simulink model "AC_motor_4"  (R2024b)
settings: Solver=FixedStepAuto  StartTime=0.0  StopTime=Tsimulation  FixedStep=Ts  RelTol=1e-3  EnableMultiTasking=on
values from neighbouring files (symbols this model uses):
  fb = 50    [AIR_Generation.m]    (also in Find_Best_Noizz.m; input_AIR80B4_3_broken_rods.m)
  J = 0.0226    [AIR_Generation.m]    (also in Find_Best_Noizz.m; input_AIR80B4_3_broken_rods.m)
  Lm = Ls - Lls    [Calculate_Basic.m]    (also in Find_Best_Noizz.m = 0.401; input_AIR80B4_3_broken_rods.m = 0.401)
  Lr = Ls    [Calculate_Basic.m]    (also in Find_Best_Noizz.m = 0.414; Run_Short_Circuit_Simulation.m = Lr*((nturns_phase-fscnturns)/nturns_phase)^2; input_AIR80B4_3_broken_rods.m = Lr*((nturns_phase-fscnturns)/nturns_phase)^2)
  Ls = 1 / 2 / pi / fb * Vph / In / (sqrt(1 - cosfi ^ 2) - cosfi * Sn / Sk)    [Calculate_Basic.m]    (also in Find_Best_Noizz.m = 0.414; Run_Short_Circuit_Simulation.m = Ls*((nturns_phase-fscnturns)/nturns_phase)^2; input_AIR80B4_3_broken_rods.m = Ls*((nturns_phase-fscnturns)/nturns_phase)^2)
  P = data{i, 2} / 2    [AIR_Generation.m]    (also in Find_Best_Noizz.m = 2; input_AIR80B4_3_broken_rods.m = 2)
  Rr = 1 / 3 * (Power + dPm) / Ikn ^ 2 / In ^2 / (1 - Sn)    [Calculate_Basic.m]    (also in Find_Best_Noizz.m = 1.274; Run_Short_Circuit_Simulation.m = Rr*((nturns_phase-fscnturns)/nturns_phase)^2; input_AIR80B4_3_broken_rods.m = Rr*((nturns_phase-fscnturns)/nturns_phase)^2)
  Rs = 1.5 * Vph ^ 2 * (1 - Sn) / C1 / (1 + C1 / Sk) / mk / (Power + dPm)    [Calculate_Basic.m]    (also in Find_Best_Noizz.m = 3.523; Run_Short_Circuit_Simulation.m = Rs*((nturns_phase-fscnturns)/nturns_phase); input_AIR80B4_3_broken_rods.m = Rs*((nturns_phase-fscnturns)/nturns_phase))
  Ts = 2e-5    (= 2e-05)    [AIR_Generation.m]    (also in Find_Best_Noizz.m; input_AIR80B4_3_broken_rods.m)
  Tswrite = 0.24e-3    (= 0.00024)    [AIR_Generation.m]    (also in Find_Best_Noizz.m; input_AIR80B4_3_broken_rods.m)
  Vph = Un / sqrt(3)    [AIR_Generation.m]    (also in Find_Best_Noizz.m = 380/sqrt(3); input_AIR80B4_3_broken_rods.m = 380/sqrt(3))
libraries: simulink x6
settings Model: Creator=srikanth  LastModifiedBy=rusla
settings SolverCC: AlgebraicLoopSolver=TrustRegion
settings DataIOCC: SignalLoggingSaveFormat=ModelDataLogs
settings OptimizationCC: ExpressionDepthLimit=2147483647  LifeSpan=inf  SimCompilerOptimization=on
settings DebuggingCC: UnderspecifiedInitializationDetection=Classic  MergeDetectMultiDrivingBlocksExec=none  FcnCallInpInsideContextMsg=warning  UnconnectedInputMsg=warning  UnconnectedOutputMsg=warning  UnconnectedLineMsg=warning  StateNameClashWarn=warning  SFUnexpectedBacktrackingDiag=warning  SFNoUnconditionalDefaultTransitionDiag=warning  SFExecutionAtInitializationDiag=none  ArithmeticOperatorsInVariantConditions=warning
settings HardwareCC: ProdBitPerPointer=32  ProdBitPerSizeT=32  ProdBitPerPtrDiffT=32  ProdLargestAtomicFloat=None  ProdIntDivRoundTo=Undefined  ProdEndianess=Unspecified  ProdWordSize=32  ProdHWDeviceType=32-bit Generic
settings ModelReferenceCC: PropagateSignalLabelsOutOfModel=off
settings SFSimCC: SimUseLocalCustomCode=off  CustomCodeUndefinedFunction=UseInterfaceOnly
settings RTWCC: RTWUseLocalCustomCode=off  GPUComputeCapability=3.5
settings CodeAppCC: StateflowObjectComments=on
settings GRTTargetCC: TargetLangStandard=C89/C90 (ANSI)  CombineOutputUpdateFcns=off  GRTInterface=on
settings ConfigComp: CovMetricSettings=dw  CovSaveCumulativeToWorkspaceVar=on  CovSaveSingleToWorkspaceVar=on  CovExternalEMLEnable=off

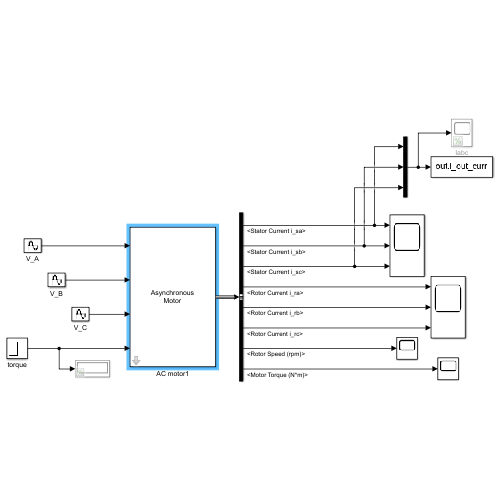
[thumbnail: Simulink's stored preview of the top-level diagram]
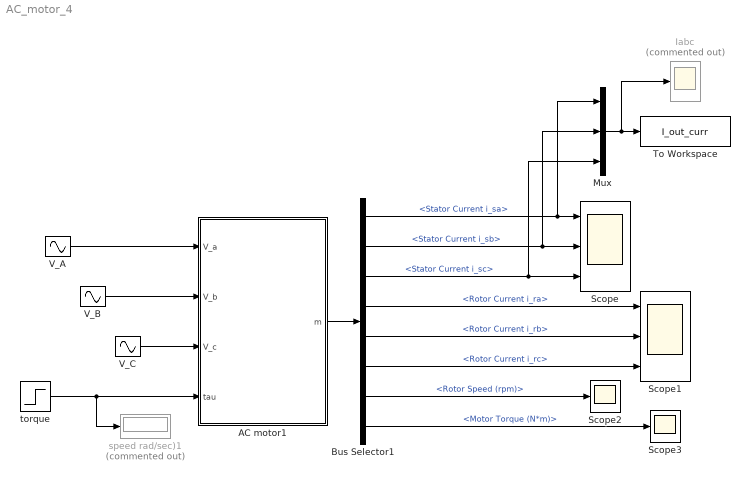
== system AC_motor_4 ==
  AC motor1 : Subsystem  mask{Rs=Rs, Ls=Ls, Rr=Rr, Lr=Lr, Lm=Lm, J=J, P=P*2}
      mask prompts: Rs "Stator Resistance  Rs [Ohm] :"; Ls "Stator Inductance Ls [H] :"; Rr "Rotor Resistance Rr [Ohm] :"; Lr "Rotor Inductance Lr [H] :"; Lm "Mutual Inductance Lm [H] :"; J "Rotor Inertia J [Kg/m^2] :"; P "Number of Poles p :"
      mask Display: fprintf('Asynchronous\nMotor')
  Bus Selector1 : BusSelector  OutputSignals=Stator.Stator Current i_sa,Stator.Stator Current i_sb,Stator.Stator Current i_sc,Rotor.Rotor Current i_ra,Rotor.Rotor Current i_rb,Rotor.Rotor Current i_rc,Mechanical.Rotor Speed (rpm),Mechanical.Motor Torque (N*m)
  Iabc : Scope  Commented=on
  Mux : Mux  Inputs=3
  Scope : Scope  NumInputPorts=3
  Scope1 : Scope  NumInputPorts=3
  Scope2 : Scope
  Scope3 : Scope
  To Workspace : ToWorkspace  VariableName=I_out_curr  SaveFormat=Structure With Time  SampleTime=Tswrite
  V_A : Sin  Amplitude=Vph  Frequency=2*pi*fb  SampleTime=Ts
  V_B : Sin  Amplitude=Vph  Frequency=2*pi*fb  Phase=-2*pi/3  SampleTime=Ts
  V_C : Sin  Amplitude=Vph  Frequency=2*pi*fb  Phase=2*pi/3  SampleTime=Ts
  speed rad/sec)1 : Display  Commented=on
  torque : Step  Time=2  After=2.3  SampleTime=0
  wires:
  torque/1 -> AC motor1/4(tau), speed rad/sec)1/1
  V_A/1 -> AC motor1/1(V_a)
  V_B/1 -> AC motor1/2(V_b)
  V_C/1 -> AC motor1/3(V_c)
  Bus Selector1/2 -> Mux/2, Scope/2  "<Stator Current i_sb>"
  Bus Selector1/3 -> Mux/3, Scope/3  "<Stator Current i_sc>"
  Bus Selector1/5 -> Scope1/2  "<Rotor Current i_rb>"
  Bus Selector1/8 -> Scope3/1  "<Motor Torque (N*m)>"
  Bus Selector1/4 -> Scope1/1  "<Rotor Current i_ra>"
  Bus Selector1/7 -> Scope2/1  "<Rotor Speed (rpm)>"
  Bus Selector1/6 -> Scope1/3  "<Rotor Current i_rc>"
  Bus Selector1/1 -> Mux/1, Scope/1  "<Stator Current i_sa>"
  Mux/1 -> Iabc/1, To Workspace/1
  AC motor1/1(m) -> Bus Selector1/1

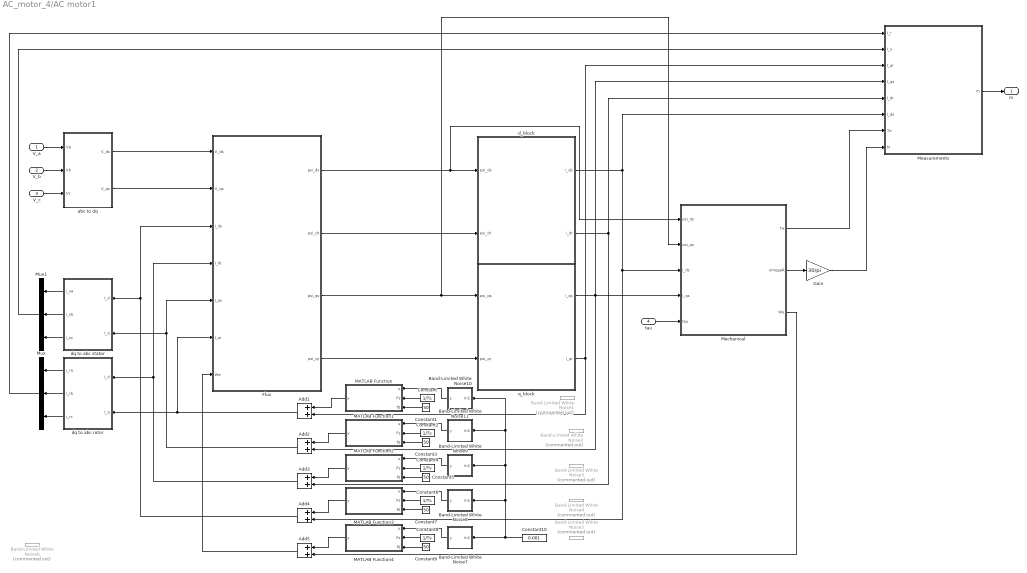
== system AC_motor_4/AC motor1 ==
  V_a : Inport
  V_b : Inport  Port=2
  V_c : Inport  Port=3
  tau : Inport  Port=4
  Add{1..5} (5 alike) : Sum
  Band-Limited White Noise1 : simulink/Sources/Band-Limited White Noise  Commented=on  Cov=[0.00001]  Ts=Ts  seed=[426526]
  Band-Limited White Noise10 : Subsystem  mask{Ts=Ts, seed=[426526]}
      mask prompts: Ts "Sample time:"
  Band-Limited White Noise11 : Subsystem  mask{Ts=Ts, seed=[921372]}
      mask prompts: Ts "Sample time:"
  Band-Limited White Noise2 : simulink/Sources/Band-Limited White Noise  Commented=on  Cov=[0.00001]  Ts=Ts  seed=[921372]
  Band-Limited White Noise3 : simulink/Sources/Band-Limited White Noise  Commented=on  Cov=[0.00001]  Ts=Ts  seed=[152264]
  Band-Limited White Noise4 : simulink/Sources/Band-Limited White Noise  Commented=on  Cov=[0.00001]  Ts=Ts  seed=[675373]
  Band-Limited White Noise5 : simulink/Sources/Band-Limited White Noise  Commented=on  Cov=[0.00001]  Ts=Ts  seed=[285858]
  Band-Limited White Noise6 : simulink/Sources/Band-Limited White Noise  Commented=on  Cov=[0.00001]  Ts=Ts  seed=[285858]
  Band-Limited White Noise7 : Subsystem  mask{Ts=Ts, seed=[285858]}
      mask prompts: Ts "Sample time:"
  Band-Limited White Noise8 : Subsystem  mask{Ts=Ts, seed=[675373]}
      mask prompts: Ts "Sample time:"
  Band-Limited White Noise9 : Subsystem  mask{Ts=Ts, seed=[152264]}
      mask prompts: Ts "Sample time:"
  Constant{,2,4,6,8} (5 alike) : Constant  Value=1/Ts
  Constant{1,3,5,7,9} (5 alike) : Constant  Value=50
  Constant10 : Constant  Value=0.001
  Flux : Subsystem
  Gain : Gain  Gain=30/pi
  MATLAB Function : MATLAB Function  TreatAsAtomicUnit=on
  MATLAB Function1 : MATLAB Function  TreatAsAtomicUnit=on
  MATLAB Function2 : MATLAB Function  TreatAsAtomicUnit=on
  MATLAB Function3 : MATLAB Function  TreatAsAtomicUnit=on
  MATLAB Function4 : MATLAB Function  TreatAsAtomicUnit=on
  Measurements : Subsystem
  Mechanical : Subsystem
  Mux : Mux  Inputs=3
  Mux1 : Mux  Inputs=3
  abc to dq : Subsystem
  d_block : Subsystem
  dq to abc rotor : Subsystem
  dq to abc stator : Subsystem
  q_block : Subsystem
  m : Outport
  wires:
  V_c/1 -> abc to dq/3(Vc)
  V_b/1 -> abc to dq/2(Vb)
  V_a/1 -> abc to dq/1(Va)
  abc to dq/1(V_ds) -> Flux/1(V_ds)
  abc to dq/2(V_qs) -> Flux/2(V_qs)
  dq to abc rotor/3(i_rc) -> Mux/3
  dq to abc rotor/1(i_ra) -> Mux/1
  dq to abc rotor/2(i_rb) -> Mux/2
  dq to abc stator/1(i_sa) -> Mux1/1
  dq to abc stator/2(i_sb) -> Mux1/2
  dq to abc stator/3(i_sc) -> Mux1/3
  Flux/3(psi_qs) -> q_block/1(psi_qs), Mechanical/2(psi_qs)
  Flux/4(psi_qr) -> q_block/2(psi_qr)
  Flux/2(psi_dr) -> d_block/2(psi_dr)
  Flux/1(psi_ds) -> d_block/1(psi_ds), Mechanical/1(psi_ds)
  tau/1 -> Mechanical/5(tau)
  q_block/1(i_qs) -> Add2/2, Measurements/4(I_qs), Mechanical/4(i_qs)
  d_block/1(i_ds) -> Add4/2, Mechanical/3(i_ds), Measurements/6(I_ds)
  Mechanical/3(We) -> Add5/2
  Mechanical/2(omegaR) -> Gain/1
  d_block/2(i_dr) -> Add3/2, Measurements/5(I_dr)
  q_block/2(i_qr) -> Add1/2, Measurements/3(I_qr)
  Measurements/1(m) -> m/1
  Gain/1 -> Measurements/8(N)
  Mechanical/1(Te) -> Measurements/7(Te)
  Mux1/1 -> Measurements/2(I_s)
  Mux/1 -> Measurements/1(I_r)
  Band-Limited White Noise10/1(y) -> MATLAB Function/1(u)
  Add1/1 -> Flux/6(I_qr), dq to abc rotor/2(I_q)
  Add2/1 -> Flux/5(I_qs), dq to abc stator/2(I_q)
  Add3/1 -> Flux/4(I_dr), dq to abc rotor/1(I_d)
  Add4/1 -> Flux/3(I_ds), dq to abc stator/1(I_d)
  Add5/1 -> Flux/7(We)
  Band-Limited White Noise11/1(y) -> MATLAB Function1/1(u)
  Band-Limited White Noise9/1(y) -> MATLAB Function2/1(u)
  Band-Limited White Noise8/1(y) -> MATLAB Function3/1(u)
  Band-Limited White Noise7/1(y) -> MATLAB Function4/1(u)
  MATLAB Function/1(y) -> Add1/1
  Constant/1 -> MATLAB Function/2(Fs)
  Constant1/1 -> MATLAB Function/3(f0)
  Constant3/1 -> MATLAB Function1/3(f0)
  Constant2/1 -> MATLAB Function1/2(Fs)
  MATLAB Function1/1(y) -> Add2/1
  Constant4/1 -> MATLAB Function2/2(Fs)
  Constant5/1 -> MATLAB Function2/3(f0)
  MATLAB Function2/1(y) -> Add3/1
  Constant7/1 -> MATLAB Function3/3(f0)
  Constant6/1 -> MATLAB Function3/2(Fs)
  MATLAB Function3/1(y) -> Add4/1
  Constant8/1 -> MATLAB Function4/2(Fs)
  Constant9/1 -> MATLAB Function4/3(f0)
  MATLAB Function4/1(y) -> Add5/1
  Constant10/1 -> Band-Limited White Noise10/1(In1), Band-Limited White Noise11/1(In1), Band-Limited White Noise9/1(In1), Band-Limited White Noise8/1(In1), Band-Limited White Noise7/1(In1)

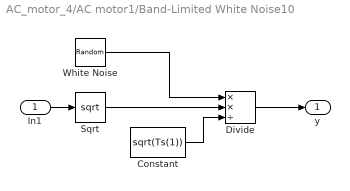
== system AC_motor_4/AC motor1/Band-Limited White Noise10 ==
  In1 : Inport
  Constant : Constant  Value=sqrt(Ts(1))
  Divide : Product  Inputs=**/
  Sqrt : Sqrt
  White Noise : RandomNumber  DisableCoverage=on  Seed=seed  SampleTime=Ts
  y : Outport
  wires:
  Sqrt/1 -> Divide/2
  In1/1 -> Sqrt/1
  Constant/1 -> Divide/3
  White Noise/1 -> Divide/1
  Divide/1 -> y/1

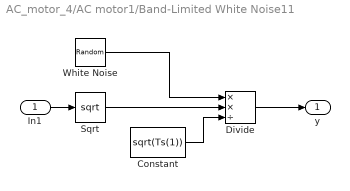
== system AC_motor_4/AC motor1/Band-Limited White Noise11 ==
  In1 : Inport
  Constant : Constant  Value=sqrt(Ts(1))
  Divide : Product  Inputs=**/
  Sqrt : Sqrt
  White Noise : RandomNumber  DisableCoverage=on  Seed=seed  SampleTime=Ts
  y : Outport
  wires:
  Divide/1 -> y/1
  White Noise/1 -> Divide/1
  Constant/1 -> Divide/3
  In1/1 -> Sqrt/1
  Sqrt/1 -> Divide/2

== system AC_motor_4/AC motor1/Band-Limited White Noise7 ==
  In1 : Inport
  Constant : Constant  Value=sqrt(Ts(1))
  Divide : Product  Inputs=**/
  Sqrt : Sqrt
  White Noise : RandomNumber  DisableCoverage=on  Seed=seed  SampleTime=Ts
  y : Outport
  wires:
  Divide/1 -> y/1
  White Noise/1 -> Divide/1
  Constant/1 -> Divide/3
  In1/1 -> Sqrt/1
  Sqrt/1 -> Divide/2

== system AC_motor_4/AC motor1/Band-Limited White Noise8 ==
  In1 : Inport
  Constant : Constant  Value=sqrt(Ts(1))
  Divide : Product  Inputs=**/
  Sqrt : Sqrt
  White Noise : RandomNumber  DisableCoverage=on  Seed=seed  SampleTime=Ts
  y : Outport
  wires:
  Sqrt/1 -> Divide/2
  In1/1 -> Sqrt/1
  Constant/1 -> Divide/3
  White Noise/1 -> Divide/1
  Divide/1 -> y/1

== system AC_motor_4/AC motor1/Band-Limited White Noise9 ==
  In1 : Inport
  Constant : Constant  Value=sqrt(Ts(1))
  Divide : Product  Inputs=**/
  Sqrt : Sqrt
  White Noise : RandomNumber  DisableCoverage=on  Seed=seed  SampleTime=Ts
  y : Outport
  wires:
  Divide/1 -> y/1
  White Noise/1 -> Divide/1
  Constant/1 -> Divide/3
  In1/1 -> Sqrt/1
  Sqrt/1 -> Divide/2

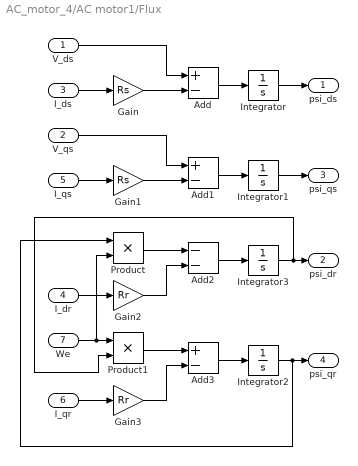
== system AC_motor_4/AC motor1/Flux ==
  V_ds : Inport
  V_qs : Inport  Port=2
  I_ds : Inport  Port=3
  I_dr : Inport  Port=4
  I_qs : Inport  Port=5
  I_qr : Inport  Port=6
  We : Inport  Port=7
  Add : Sum  Inputs=+-
  Add1 : Sum  Inputs=+-
  Add2 : Sum  Inputs=--
  Add3 : Sum  Inputs=+-
  Gain : Gain  Gain=Rs
  Gain1 : Gain  Gain=Rs
  Gain2 : Gain  Gain=Rr
  Gain3 : Gain  Gain=Rr
  Integrator{,1..3} (4 alike) : Integrator
  Product : Product
  Product1 : Product
  psi_ds : Outport
  psi_dr : Outport  Port=2
  psi_qs : Outport  Port=3
  psi_qr : Outport  Port=4
  wires:
  I_ds/1 -> Gain/1
  Gain/1 -> Add/2
  V_ds/1 -> Add/1
  Add/1 -> Integrator/1
  Integrator/1 -> psi_ds/1
  V_qs/1 -> Add1/1
  Gain1/1 -> Add1/2
  I_qs/1 -> Gain1/1
  Add1/1 -> Integrator1/1
  Integrator1/1 -> psi_qs/1
  Integrator2/1 -> Product/1, psi_qr/1
  Integrator3/1 -> Product1/2, psi_dr/1
  Add2/1 -> Integrator3/1
  Product/1 -> Add2/1
  I_dr/1 -> Gain2/1
  I_qr/1 -> Gain3/1
  Gain2/1 -> Add2/2
  We/1 -> Product/2, Product1/1
  Product1/1 -> Add3/1
  Gain3/1 -> Add3/2
  Add3/1 -> Integrator2/1

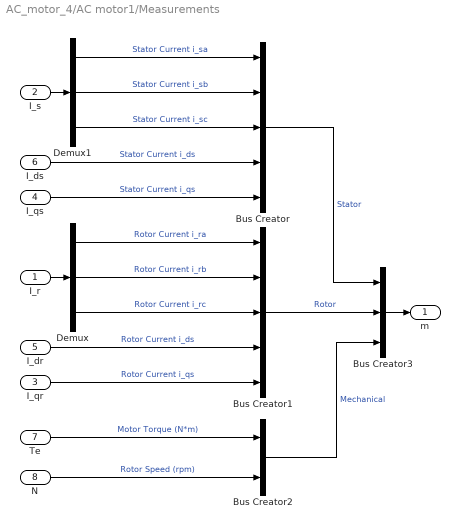
== system AC_motor_4/AC motor1/Measurements ==
  I_r : Inport
  I_s : Inport  Port=2
  I_qr : Inport  Port=3
  I_qs : Inport  Port=4
  I_dr : Inport  Port=5
  I_ds : Inport  Port=6
  Te : Inport  Port=7
  N : Inport  Port=8
  Bus Creator : BusCreator  Inputs=5
  Bus Creator1 : BusCreator  Inputs=5
  Bus Creator2 : BusCreator  Inputs=2
  Bus Creator3 : BusCreator  Inputs=3
  Demux : Demux  Outputs=3
  Demux1 : Demux  Outputs=3
  m : Outport
  wires:
  Bus Creator3/1 -> m/1
  Bus Creator/1 -> Bus Creator3/1  "Stator"
  Bus Creator1/1 -> Bus Creator3/2  "Rotor"
  Bus Creator2/1 -> Bus Creator3/3  "Mechanical"
  Te/1 -> Bus Creator2/1  "Motor Torque (N*m)"
  N/1 -> Bus Creator2/2  "Rotor Speed (rpm)"
  I_dr/1 -> Bus Creator1/4  "Rotor Current i_ds"
  I_qr/1 -> Bus Creator1/5  "Rotor Current i_qs"
  Demux/2 -> Bus Creator1/2  "Rotor Current i_rb"
  Demux/1 -> Bus Creator1/1  "Rotor Current i_ra"
  Demux/3 -> Bus Creator1/3  "Rotor Current i_rc"
  I_r/1 -> Demux/1
  Demux1/1 -> Bus Creator/1  "Stator Current i_sa"
  Demux1/2 -> Bus Creator/2  "Stator Current i_sb"
  Demux1/3 -> Bus Creator/3  "Stator Current i_sc"
  I_ds/1 -> Bus Creator/4  "Stator Current i_ds"
  I_qs/1 -> Bus Creator/5  "Stator Current i_qs"
  I_s/1 -> Demux1/1

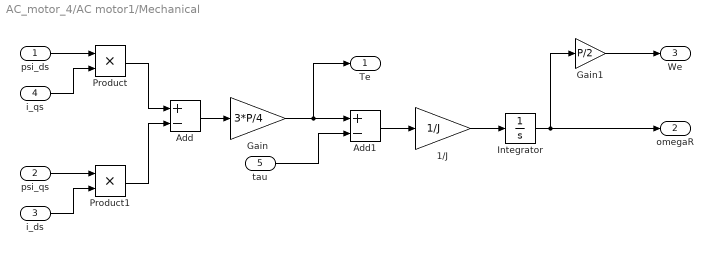
== system AC_motor_4/AC motor1/Mechanical ==
  psi_ds : Inport
  psi_qs : Inport  Port=2
  i_ds : Inport  Port=3
  i_qs : Inport  Port=4
  tau : Inport  Port=5
  1/J : Gain  Gain=1/J
  Add : Sum  Inputs=+-
  Add1 : Sum  Inputs=+-
  Gain : Gain  Gain=3*P/4
  Gain1 : Gain  Gain=P/2
  Integrator : Integrator
  Product : Product
  Product1 : Product
  Te : Outport
  omegaR : Outport  Port=2
  We : Outport  Port=3
  wires:
  psi_ds/1 -> Product/1
  i_qs/1 -> Product/2
  psi_qs/1 -> Product1/1
  i_ds/1 -> Product1/2
  Product/1 -> Add/1
  Product1/1 -> Add/2
  Add/1 -> Gain/1
  Gain/1 -> Add1/1, Te/1
  tau/1 -> Add1/2
  Add1/1 -> 1/J/1
  1/J/1 -> Integrator/1
  Gain1/1 -> We/1
  Integrator/1 -> Gain1/1, omegaR/1

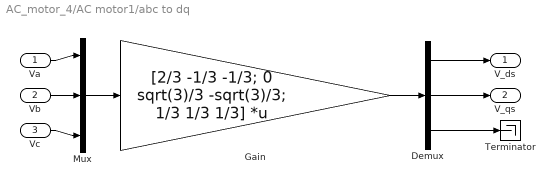
== system AC_motor_4/AC motor1/abc to dq ==
  Va : Inport
  Vb : Inport  Port=2
  Vc : Inport  Port=3
  Demux : Demux  Outputs=3
  Gain : Gain  Gain=[2/3 -1/3 -1/3; 0 sqrt(3)/3 -sqrt(3)/3; 1/3 1/3 1/3]  Multiplication=Matrix(K*u)
  Mux : Mux  Inputs=3
  Terminator : Terminator
  V_ds : Outport
  V_qs : Outport  Port=2
  wires:
  Va/1 -> Mux/1
  Vb/1 -> Mux/2
  Vc/1 -> Mux/3
  Mux/1 -> Gain/1
  Gain/1 -> Demux/1
  Demux/3 -> Terminator/1
  Demux/1 -> V_ds/1
  Demux/2 -> V_qs/1

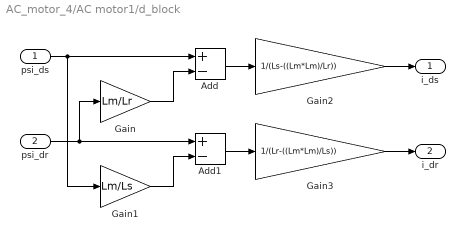
== system AC_motor_4/AC motor1/d_block ==
  psi_ds : Inport
  psi_dr : Inport  Port=2
  Add : Sum  Inputs=+-
  Add1 : Sum  Inputs=+-
  Gain : Gain  Gain=Lm/Lr
  Gain1 : Gain  Gain=Lm/Ls
  Gain2 : Gain  Gain=1/(Ls-((Lm*Lm)/Lr))
  Gain3 : Gain  Gain=1/(Lr-((Lm*Lm)/Ls))
  i_ds : Outport
  i_dr : Outport  Port=2
  wires:
  psi_ds/1 -> Add/1, Gain1/1
  Gain/1 -> Add/2
  Gain1/1 -> Add1/2
  psi_dr/1 -> Gain/1, Add1/1
  Gain2/1 -> i_ds/1
  Add/1 -> Gain2/1
  Add1/1 -> Gain3/1
  Gain3/1 -> i_dr/1

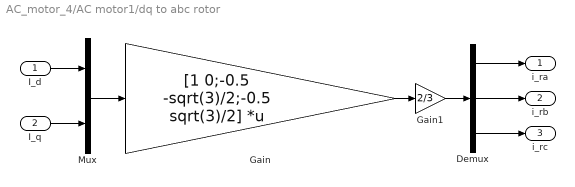
== system AC_motor_4/AC motor1/dq to abc rotor ==
  I_d : Inport
  I_q : Inport  Port=2
  Demux : Demux  Outputs=3
  Gain : Gain  Gain=[1 0;-0.5 -sqrt(3)/2;-0.5 sqrt(3)/2]  Multiplication=Matrix(K*u)
  Gain1 : Gain  Gain=2/3
  Mux : Mux  Inputs=2
  i_ra : Outport
  i_rb : Outport  Port=2
  i_rc : Outport  Port=3
  wires:
  Gain/1 -> Gain1/1
  Demux/1 -> i_ra/1
  I_q/1 -> Mux/2
  Demux/2 -> i_rb/1
  Mux/1 -> Gain/1
  I_d/1 -> Mux/1
  Gain1/1 -> Demux/1
  Demux/3 -> i_rc/1

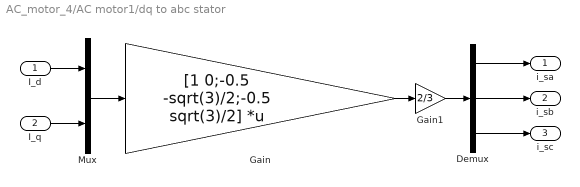
== system AC_motor_4/AC motor1/dq to abc stator ==
  I_d : Inport
  I_q : Inport  Port=2
  Demux : Demux  Outputs=3
  Gain : Gain  Gain=[1 0;-0.5 -sqrt(3)/2;-0.5 sqrt(3)/2]  Multiplication=Matrix(K*u)
  Gain1 : Gain  Gain=2/3
  Mux : Mux  Inputs=2
  i_sa : Outport
  i_sb : Outport  Port=2
  i_sc : Outport  Port=3
  wires:
  Demux/2 -> i_sb/1
  Demux/3 -> i_sc/1
  I_q/1 -> Mux/2
  I_d/1 -> Mux/1
  Demux/1 -> i_sa/1
  Mux/1 -> Gain/1
  Gain/1 -> Gain1/1
  Gain1/1 -> Demux/1

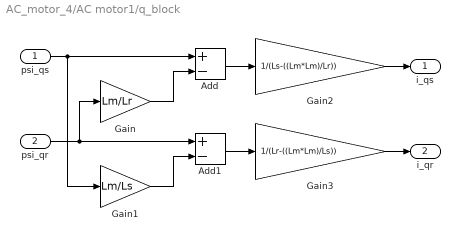
== system AC_motor_4/AC motor1/q_block ==
  psi_qs : Inport
  psi_qr : Inport  Port=2
  Add : Sum  Inputs=+-
  Add1 : Sum  Inputs=+-
  Gain : Gain  Gain=Lm/Lr
  Gain1 : Gain  Gain=Lm/Ls
  Gain2 : Gain  Gain=1/(Ls-((Lm*Lm)/Lr))
  Gain3 : Gain  Gain=1/(Lr-((Lm*Lm)/Ls))
  i_qs : Outport
  i_qr : Outport  Port=2
  wires:
  Gain/1 -> Add/2
  Gain3/1 -> i_qr/1
  psi_qs/1 -> Add/1, Gain1/1
  Gain2/1 -> i_qs/1
  Add1/1 -> Gain3/1
  psi_qr/1 -> Gain/1, Add1/1
  Gain1/1 -> Add1/2
  Add/1 -> Gain2/1

== matlab function AC_motor_4/AC motor1/MATLAB Function ==
  data: u input; y output; Fs input; f0 input
function y = colored_noise(u, Fs, f0)
%#codegen
% u    : input white noise sample (scalar)
% fs   : sample rate (Hz)
% f0   : target frequency (Hz), 0 < f0 < fs/2
% bw   : 3-dB bandwidth around f0 (Hz), small positive number
% gain : linear gain at the peak (~ amplitude scaling). Use 1.0 if unsure.
%
% y    : output noise sample, shaped to increase near f0
bw = 5;
gain = 1;

persistent b a zi prev_Fs prev_f0 prev_bw prev_gain init
if isempty(init)
    [b,a] = designPeakNorm(Fs,f0,bw,gain);
    zi = zeros(max(numel(a),numel(b)) - 1, 1);
    prev_Fs=Fs; prev_f0=f0; prev_bw=bw; prev_gain=gain; init=true;
end

if Fs~=prev_Fs || f0~=prev_f0 || bw~=prev_bw || gain~=prev_gain
    [b,a] = designPeakNorm(Fs,f0,bw,gain);
    zi = zeros(max(numel(a),numel(b)) - 1, 1);
    prev_Fs=Fs; prev_f0=f0; prev_bw=bw; prev_gain=gain;
end

[y, zi] = filter(b, a, u, zi);
end

function [b,a] = designPeakNorm(Fs,f0,bw,gain)
% Clamp for stability and validity
epsv = 1e-6;
Fs    = max(Fs, epsv);
f0    = min(max(f0, epsv), Fs/2 - epsv);
bwMax = min(f0 - epsv, Fs/2 - f0 - epsv);
bw    = min(max(bw, epsv), max(bwMax, epsv));

% Normalize to Nyquist
Wo = f0 / (Fs/2);   % 0<Wo<1
BW = bw / (Fs/2);   % 0<BW<1

% Peaking IIR (normalized form)
[b,a] = iirpeak(Wo, BW);

% Set peak gain
b = b * gain;
end

== matlab function AC_motor_4/AC motor1/MATLAB Function2 ==
  data: u input; y output; Fs input; f0 input
function y = colored_noise(u, Fs, f0)
%#codegen
% u    : input white noise sample (scalar)
% fs   : sample rate (Hz)
% f0   : target frequency (Hz), 0 < f0 < fs/2
% bw   : 3-dB bandwidth around f0 (Hz), small positive number
% gain : linear gain at the peak (~ amplitude scaling). Use 1.0 if unsure.
%
% y    : output noise sample, shaped to increase near f0
bw = 5;
gain = 1;

persistent b a zi prev_Fs prev_f0 prev_bw prev_gain init
if isempty(init)
    [b,a] = designPeakNorm(Fs,f0,bw,gain);
    zi = zeros(max(numel(a),numel(b)) - 1, 1);
    prev_Fs=Fs; prev_f0=f0; prev_bw=bw; prev_gain=gain; init=true;
end

if Fs~=prev_Fs || f0~=prev_f0 || bw~=prev_bw || gain~=prev_gain
    [b,a] = designPeakNorm(Fs,f0,bw,gain);
    zi = zeros(max(numel(a),numel(b)) - 1, 1);
    prev_Fs=Fs; prev_f0=f0; prev_bw=bw; prev_gain=gain;
end

[y, zi] = filter(b, a, u, zi);
end

function [b,a] = designPeakNorm(Fs,f0,bw,gain)
% Clamp for stability and validity
epsv = 1e-6;
Fs    = max(Fs, epsv);
f0    = min(max(f0, epsv), Fs/2 - epsv);
bwMax = min(f0 - epsv, Fs/2 - f0 - epsv);
bw    = min(max(bw, epsv), max(bwMax, epsv));

% Normalize to Nyquist
Wo = f0 / (Fs/2);   % 0<Wo<1
BW = bw / (Fs/2);   % 0<BW<1

% Peaking IIR (normalized form)
[b,a] = iirpeak(Wo, BW);

% Set peak gain
b = b * gain;
end

== matlab function AC_motor_4/AC motor1/MATLAB Function3 ==
  data: u input; y output; Fs input; f0 input
function y = colored_noise(u, Fs, f0)
%#codegen
% u    : input white noise sample (scalar)
% fs   : sample rate (Hz)
% f0   : target frequency (Hz), 0 < f0 < fs/2
% bw   : 3-dB bandwidth around f0 (Hz), small positive number
% gain : linear gain at the peak (~ amplitude scaling). Use 1.0 if unsure.
%
% y    : output noise sample, shaped to increase near f0
bw = 5;
gain = 1;

persistent b a zi prev_Fs prev_f0 prev_bw prev_gain init
if isempty(init)
    [b,a] = designPeakNorm(Fs,f0,bw,gain);
    zi = zeros(max(numel(a),numel(b)) - 1, 1);
    prev_Fs=Fs; prev_f0=f0; prev_bw=bw; prev_gain=gain; init=true;
end

if Fs~=prev_Fs || f0~=prev_f0 || bw~=prev_bw || gain~=prev_gain
    [b,a] = designPeakNorm(Fs,f0,bw,gain);
    zi = zeros(max(numel(a),numel(b)) - 1, 1);
    prev_Fs=Fs; prev_f0=f0; prev_bw=bw; prev_gain=gain;
end

[y, zi] = filter(b, a, u, zi);
end

function [b,a] = designPeakNorm(Fs,f0,bw,gain)
% Clamp for stability and validity
epsv = 1e-6;
Fs    = max(Fs, epsv);
f0    = min(max(f0, epsv), Fs/2 - epsv);
bwMax = min(f0 - epsv, Fs/2 - f0 - epsv);
bw    = min(max(bw, epsv), max(bwMax, epsv));

% Normalize to Nyquist
Wo = f0 / (Fs/2);   % 0<Wo<1
BW = bw / (Fs/2);   % 0<BW<1

% Peaking IIR (normalized form)
[b,a] = iirpeak(Wo, BW);

% Set peak gain
b = b * gain;
end

== matlab function AC_motor_4/AC motor1/MATLAB Function4 ==
  data: u input; y output; Fs input; f0 input
function y = colored_noise(u, Fs, f0)
%#codegen
% u    : input white noise sample (scalar)
% fs   : sample rate (Hz)
% f0   : target frequency (Hz), 0 < f0 < fs/2
% bw   : 3-dB bandwidth around f0 (Hz), small positive number
% gain : linear gain at the peak (~ amplitude scaling). Use 1.0 if unsure.
%
% y    : output noise sample, shaped to increase near f0
bw = 5;
gain = 1;

persistent b a zi prev_Fs prev_f0 prev_bw prev_gain init
if isempty(init)
    [b,a] = designPeakNorm(Fs,f0,bw,gain);
    zi = zeros(max(numel(a),numel(b)) - 1, 1);
    prev_Fs=Fs; prev_f0=f0; prev_bw=bw; prev_gain=gain; init=true;
end

if Fs~=prev_Fs || f0~=prev_f0 || bw~=prev_bw || gain~=prev_gain
    [b,a] = designPeakNorm(Fs,f0,bw,gain);
    zi = zeros(max(numel(a),numel(b)) - 1, 1);
    prev_Fs=Fs; prev_f0=f0; prev_bw=bw; prev_gain=gain;
end

[y, zi] = filter(b, a, u, zi);
end

function [b,a] = designPeakNorm(Fs,f0,bw,gain)
% Clamp for stability and validity
epsv = 1e-6;
Fs    = max(Fs, epsv);
f0    = min(max(f0, epsv), Fs/2 - epsv);
bwMax = min(f0 - epsv, Fs/2 - f0 - epsv);
bw    = min(max(bw, epsv), max(bwMax, epsv));

% Normalize to Nyquist
Wo = f0 / (Fs/2);   % 0<Wo<1
BW = bw / (Fs/2);   % 0<BW<1

% Peaking IIR (normalized form)
[b,a] = iirpeak(Wo, BW);

% Set peak gain
b = b * gain;
end

== matlab function AC_motor_4/AC motor1/MATLAB Function1 ==
  data: u input; y output; Fs input; f0 input
function y = colored_noise(u, Fs, f0)
%#codegen
% u    : input white noise sample (scalar)
% fs   : sample rate (Hz)
% f0   : target frequency (Hz), 0 < f0 < fs/2
% bw   : 3-dB bandwidth around f0 (Hz), small positive number
% gain : linear gain at the peak (~ amplitude scaling). Use 1.0 if unsure.
%
% y    : output noise sample, shaped to increase near f0
bw = 5;
gain = 1;

persistent b a zi prev_Fs prev_f0 prev_bw prev_gain init
if isempty(init)
    [b,a] = designPeakNorm(Fs,f0,bw,gain);
    zi = zeros(max(numel(a),numel(b)) - 1, 1);
    prev_Fs=Fs; prev_f0=f0; prev_bw=bw; prev_gain=gain; init=true;
end

if Fs~=prev_Fs || f0~=prev_f0 || bw~=prev_bw || gain~=prev_gain
    [b,a] = designPeakNorm(Fs,f0,bw,gain);
    zi = zeros(max(numel(a),numel(b)) - 1, 1);
    prev_Fs=Fs; prev_f0=f0; prev_bw=bw; prev_gain=gain;
end

[y, zi] = filter(b, a, u, zi);
end

function [b,a] = designPeakNorm(Fs,f0,bw,gain)
% Clamp for stability and validity
epsv = 1e-6;
Fs    = max(Fs, epsv);
f0    = min(max(f0, epsv), Fs/2 - epsv);
bwMax = min(f0 - epsv, Fs/2 - f0 - epsv);
bw    = min(max(bw, epsv), max(bwMax, epsv));

% Normalize to Nyquist
Wo = f0 / (Fs/2);   % 0<Wo<1
BW = bw / (Fs/2);   % 0<BW<1

% Peaking IIR (normalized form)
[b,a] = iirpeak(Wo, BW);

% Set peak gain
b = b * gain;
end
